simulink model "Dynamics"  (R2017a)
settings: Solver=VariableStepAuto  StartTime=0.0  StopTime=100  RelTol=1e-3
(part 8 of 8)

== matlab function Dynamics/omega ==
  data: q input; wx output; qd input; wy output; wz output
function [wx ,wy, wz] = fcn(q , qd)

q1 = q(1);
q2 = q(2);
q3 = q(3);
q4 = q(4);
q5 = q(5);
q6 = q(6);

c1 = cos(q(1));
c2 = cos(q(2));
c3 = cos(q(3));
c4 = cos(q(4));
c5 = cos(q(5));
c6 = cos(q(6));
s1 = sin(q(1));
s2 = sin(q(2));
s3 = sin(q(3));
s4 = sin(q(4));
s5 = sin(q(5));
s6 = sin(q(6));

wx = c6*(c5*(-c3*s4*(q(1) + q(2)) + c4*s3*(q(1) + q(2))) - s5*(-q(3) + q(4))) - s6*(-c5*(-q(3) + q(4)) - s5*(-c3*s4*(q(1) + q(2)) + c4*s3*(q(1) + q(2))));
  
wy = -c6*(-c5*(-q(3) + q(4)) - s5*(-c3*s4*(q(1) + q(2)) + c4*s3*(q(1) + q(2)))) - s6*(c5*(-c3*s4*(q(1) + q(2)) + c4*s3*(q(1) + q(2))) - s5*(-q(3) + q(4)));
  
wz = c3*c4*(q(1) + q(2)) - q(5) + q(6) + s3*s4*(q(1) + q(2));

== matlab function Dynamics/POSITION ==
  data: q input; px output; py output; pz output
function [px,py,pz] = fcn(q)
%#codegen

q1 = q(1);
q2 = q(2);
q3 = q(3);
q4 = q(4);
q5 = q(5);
q6 = q(6);


px = 270*cos(q(1)) + 90*cos(q(1))*cos(q(2)) - 295*cos(q(1))*sin(q(2)) - 295*cos(q(2))*sin(q(1)) - 90*sin(q(1))*sin(q(2)) + 80*cos(q(3))*sin(q(4))*(cos(q(1))*cos(q(2)) - sin(q(1))*sin(q(2))) - 80*cos(q(4))*sin(q(3))*(cos(q(1))*cos(q(2)) - sin(q(1))*sin(q(2))) + 75;
py = 80*cos(q(3))*cos(q(4)) + 80*sin(q(3))*sin(q(4)) + 335;
pz = 295*sin(q(1))*sin(q(2)) - 295*cos(q(1))*cos(q(2)) - 90*cos(q(1))*sin(q(2)) - 90*cos(q(2))*sin(q(1)) - 270*sin(q(1)) - 80*cos(q(3))*sin(q(4))*(cos(q(1))*sin(q(2)) + cos(q(2))*sin(q(1))) + 80*cos(q(4))*sin(q(3))*(cos(q(1))*sin(q(2)) + cos(q(2))*sin(q(1)));
 

 px;
 py;
 pz

== matlab function Dynamics/omegadot ==
  data: q input; wdotx output; qd input; wdoty output; wdotz output; qdd input
function [wdotx ,wdoty, wdotz] = fcn(q , qd, qdd)

q1 = q(1);
q2 = q(2);
q3 = q(3);
q4 = q(4);
q5 = q(5);
q6 = q(6);

c1 = cos(q(1));
c2 = cos(q(2));
c3 = cos(q(3));
c4 = cos(q(4));
c5 = cos(q(5));
c6 = cos(q(6));
s1 = sin(q(1));
s2 = sin(q(2));
s3 = sin(q(3));
s4 = sin(q(4));
s5 = sin(q(5));
s6 = sin(q(6));

wdotx = c6*(c5*(c4*(c3*qd(3)*(qd(1) + qd(2)) + s3*(qdd(1) + qdd(2))) + qd(4)*(-c3*c4*(qd(1) + qd(2)) - s3*s4*(qd(1) + qd(2))) - s4*(c3*(qdd(1) + qdd(2)) - qd(3)*s3*(qd(1) + qd(2)))) + qd(5)*(-c5*(-qd(3) + qd(4)) - s5*(-c3*s4*(qd(1) + qd(2)) + c4*s3*(qd(1) + qd(2)))) - s5*(-qdd(3) + qdd(4))) + qd(6)*(-c6*(-c5*(-qd(3) + qd(4)) - s5*(-c3*s4*(qd(1) + qd(2)) + c4*s3*(qd(1) + qd(2)))) - s6*(c5*(-c3*s4*(qd(1) + qd(2)) + c4*s3*(qd(1) + qd(2))) - s5*(-qd(3) + qd(4)))) - s6*(-c5*(-qdd(3) + qdd(4)) - qd(5)*(c5*(-c3*s4*(qd(1) + qd(2)) + c4*s3*(qd(1) + qd(2))) - s5*(-qd(3) + qd(4))) - s5*(c4*(c3*qd(3)*(qd(1) + qd(2)) + s3*(qdd(1) + qdd(2))) + qd(4)*(-c3*c4*(qd(1) + qd(2)) - s3*s4*(qd(1) + qd(2))) - s4*(c3*(qdd(1) + qdd(2)) - qd(3)*s3*(qd(1) + qd(2)))));
wdoty = -c6*(-c5*(-qdd(3) + qdd(4)) - qd(5)*(c5*(-c3*s4*(qd(1) + qd(2)) + c4*s3*(qd(1) + qd(2))) - s5*(-qd(3) + qd(4))) - s5*(c4*(c3*qd(3)*(qd(1) + qd(2)) + s3*(qdd(1) + qdd(2))) + qd(4)*(-c3*c4*(qd(1) + qd(2)) - s3*s4*(qd(1) + qd(2))) - s4*(c3*(qdd(1) + qdd(2)) - qd(3)*s3*(qd(1) + qd(2))))) - qd(6)*(c6*(c5*(-c3*s4*(qd(1) + qd(2)) + c4*s3*(qd(1) + qd(2))) - s5*(-qd(3) + qd(4))) - s6*(-c5*(-qd(3) + qd(4)) - s5*(-c3*s4*(qd(1) + qd(2)) + c4*s3*(qd(1) + qd(2))))) - s6*(c5*(c4*(c3*qd(3)*(qd(1) + qd(2)) + s3*(qdd(1) + qdd(2))) + qd(4)*(-c3*c4*(qd(1) + qd(2)) - s3*s4*(qd(1) + qd(2))) - s4*(c3*(qdd(1) + qdd(2)) - qd(3)*s3*(qd(1) + qd(2)))) + qd(5)*(-c5*(-qd(3) + qd(4)) - s5*(-c3*s4*(qd(1) + qd(2)) + c4*s3*(qd(1) + qd(2)))) - s5*(-qdd(3) + qdd(4)));
  
wdotz = c4*(c3*(qdd(1) + qdd(2)) - qd(3)*s3*(qd(1) + qd(2))) + qd(4)*(-c3*s4*(qd(1) + qd(2)) + c4*s3*(qd(1) + qd(2))) - qdd(5) + qdd(6) + s4*(c3*qd(3)*(qd(1) + qd(2)) + s3*(qdd(1) + qdd(2)));
